simulink model "pcm_giaidieubien"  (R2023a)
settings: Solver=VariableStepAuto  StartTime=0.0  StopTime=1  RelTol=1e-3
libraries: simulink x2, dspquant2 x2, dspfdesign x1, dspsigops x1
settings Model: Creator=dung  LastModifiedBy=dung

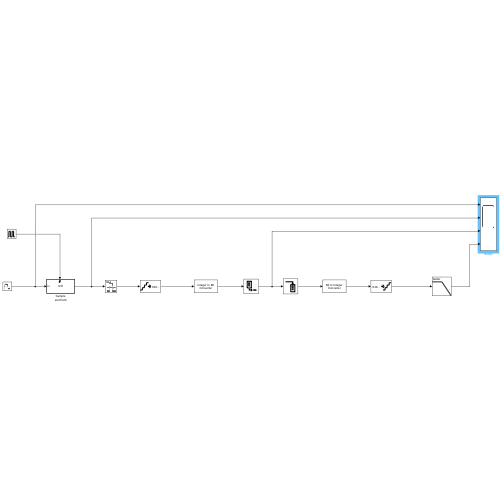
[thumbnail: Simulink's stored preview of the top-level diagram]
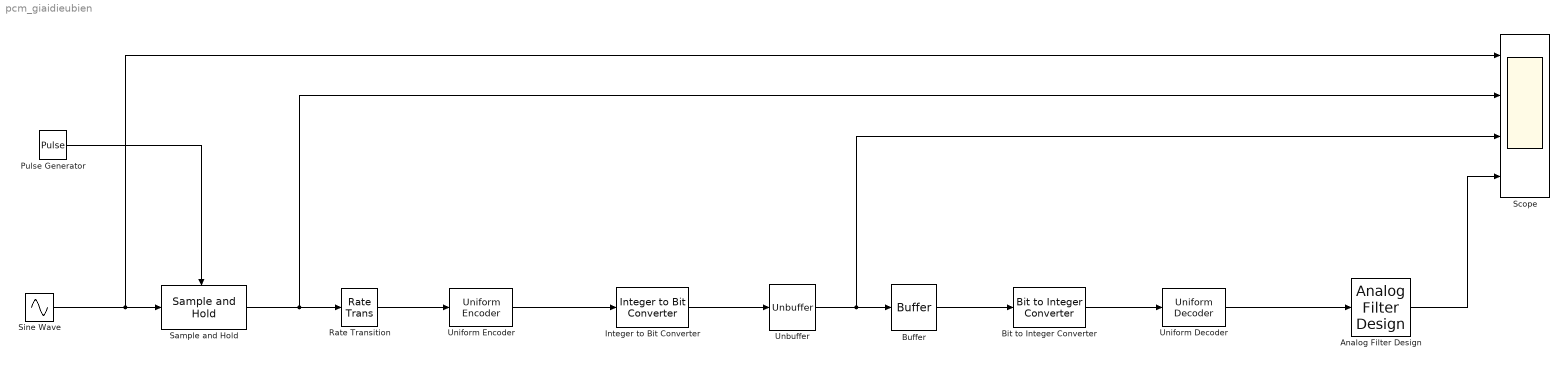
== system pcm_giaidieubien ==
  Analog Filter Design : dspfdesign/Analog Filter Design  method=Butterworth  filttype=Lowpass  N=12  Wlo=2*pi*3100  Whi=80  Rp=2  Rs=40
  Bit to Integer Converter : simulink/Logic and Bit Operations/Bit to Integer Converter  nbits=8  bitOrder=MSB first  signedOutputValues=Unsigned  outDtype=Inherit via internal rule  outDtypeSigned=Inherit via internal rule
  Buffer : Buffer  N=8  OutputFrames=off
  Integer to Bit Converter : simulink/Logic and Bit Operations/Integer to Bit Converter  nbits=8  signedInputValues=Unsigned  bitOrder=MSB first  outDtype=Inherit via internal rule
  Pulse Generator : DiscretePulseGenerator  PulseType=Time based  Period=1/8000  PulseWidth=50
  Rate Transition : RateTransition  OutPortSampleTime=1/8000
  Sample and Hold : dspsigops/Sample and Hold  trig=Rising edge  initCond=0  latchinput=off
  Scope : Scope  NumInputPorts=4
  Sine Wave : Sin  Frequency=2*pi*3000  SampleTime=1/64000
  Unbuffer : Unbuffer
  Uniform Decoder : dspquant2/Uniform Decoder  peak=1  bits=8  overflowMode=Saturate  otype=Double
  Uniform Encoder : dspquant2/Uniform Encoder  peak=1  bits=8  otype=Unsigned integer
  wires:
  Uniform Encoder/1 -> Integer to Bit Converter/1
  Sample and Hold/1 -> Scope/2, Rate Transition/1
  Sine Wave/1 -> Scope/1, Sample and Hold/1
  Rate Transition/1 -> Uniform Encoder/1
  Integer to Bit Converter/1 -> Unbuffer/1
  Pulse Generator/1 -> Sample and Hold/Trigger
  Unbuffer/1 -> Scope/3, Buffer/1
  Buffer/1 -> Bit to Integer Converter/1
  Bit to Integer Converter/1 -> Uniform Decoder/1
  Uniform Decoder/1 -> Analog Filter Design/1
  Analog Filter Design/1 -> Scope/4
